simulink model "ActiveBalancingModelling"  (R2024b)
settings: Solver=FixedStepAuto  StartTime=0.0  StopTime=1000  FixedStep=SampleTime  RelTol=1e-3
model workspace (MAT data in the model file):
  Ah = 3
  C = 0.001
  R = 0.001
  SampleTime = 0.0001
  SoC1 = 60
  SoC2 = 70
  SoC3 = 50
  SoC4 = 80
  Vnom = 3.7
undefined symbols (not defined in the file or in its folder): Ion, Lithium
libraries: spsIdealSwitchLib x8, spsSeriesRLCBranchLib x5, spsBatteryLib x4, sps_lib x1
settings Model: Creator=MOHAMED  LastModifiedBy=MOHAMED

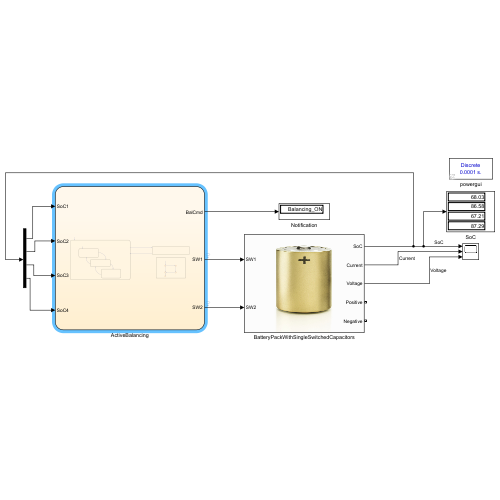
[thumbnail: Simulink's stored preview of the top-level diagram]
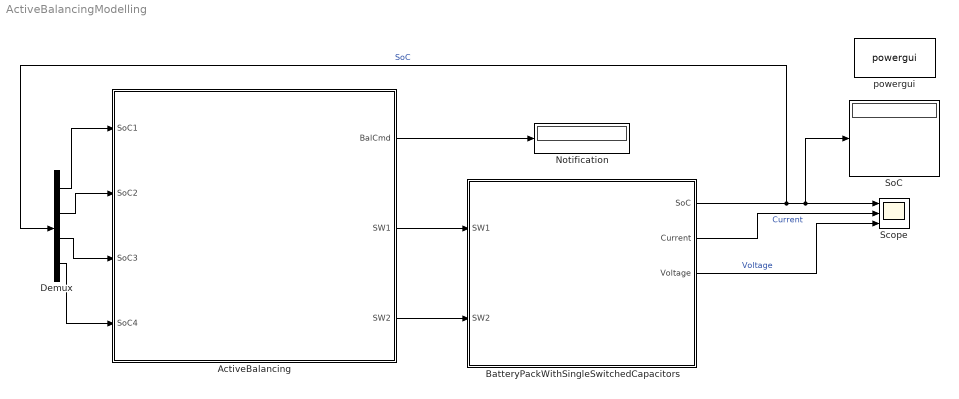
== system ActiveBalancingModelling ==
  ActiveBalancing : Stateflow chart  TreatAsAtomicUnit=on
  BatteryPackWithSingleSwitchedCapacitors : Subsystem
      mask Display: image('battery.jpg');
  Demux : Demux
  Notification : Display
  Scope : Scope  NumInputPorts=3
  SoC : Display
  powergui : sps_lib/powergui  Priority=1  SimulationMode=Discrete  SampleTime=SampleTime  frequency=60  Iterations=50  frequencyindice=0  Pbase=100e6  ErrMax=1e-4  UnitsV=kV  UnitsW=MW  buscounter=0  FunctionMessages=off  echomessages=off  EnableUseOfTLC=off  CurrentSourceSwitches=off  DisableSnubberDevices=off  DisableRonSwitches=off  DisableVfSwitches=off  DisplayEquations=off  AutomaticDiscreteSolvers=off  SolverType=Tustin/Backward Euler (TBE)  Interpol=off  ExternalGateDelay=off  methode=off  Ts=100  x0status=blocks  SPID=on  SwTol=0  HookPort=off  NonlinearTolerance=1e-4  nMaxIteration=100  ContinueOnMaxIteration=off  RestoreLinks=warning  ResistiveCurrentMeasurement=off  Frange=[0:2:500]  Ylog=off  Xlog=on  ShowGrid=off  save=off  variable=ZData  structure=0  ZoomFFT=off  StartTime=0.0  cycles=1  DisplayStyle=1  fundamental=60  FreqAxis=off  MaxFrequency=1000  frequencyindicesteady=1  RmsSteady=1  display=off
  wires:
  BatteryPackWithSingleSwitchedCapacitors/1(SoC) -> Demux/1, SoC/1, Scope/1  "SoC"
  BatteryPackWithSingleSwitchedCapacitors/2(Current) -> Scope/2  "Current"
  BatteryPackWithSingleSwitchedCapacitors/3(Voltage) -> Scope/3  "Voltage"
  ActiveBalancing/1(BalCmd) -> Notification/1
  ActiveBalancing/2(SW1) -> BatteryPackWithSingleSwitchedCapacitors/1(SW1)
  ActiveBalancing/3(SW2) -> BatteryPackWithSingleSwitchedCapacitors/2(SW2)
  Demux/1 -> ActiveBalancing/1(SoC1)
  Demux/2 -> ActiveBalancing/2(SoC2)
  Demux/3 -> ActiveBalancing/3(SoC3)
  Demux/4 -> ActiveBalancing/4(SoC4)

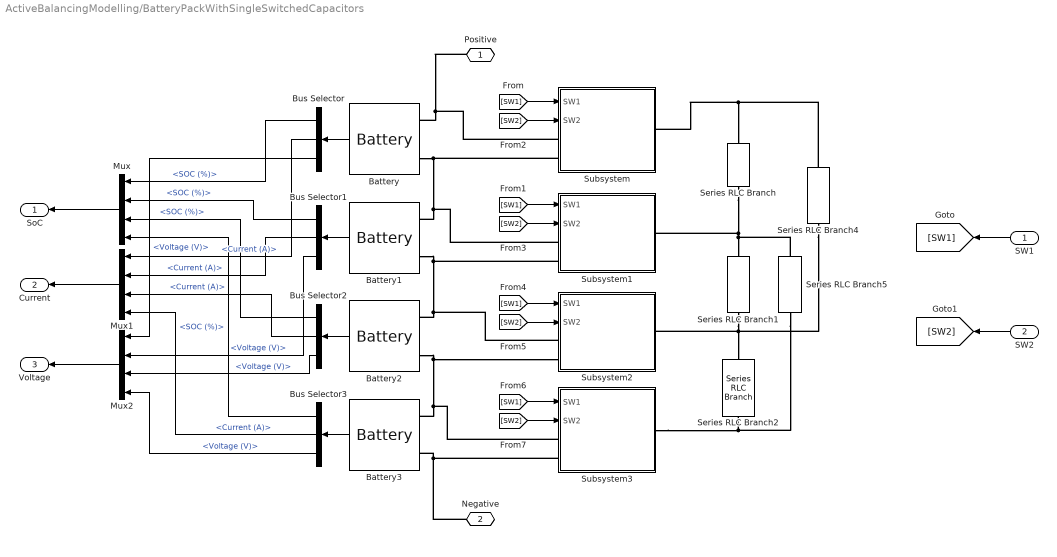
== system ActiveBalancingModelling/BatteryPackWithSingleSwitchedCapacitors ==
  SW1 : Inport
  SW2 : Inport  Port=2
  Battery : spsBatteryLib/Battery  BatType=Lithium-Ion  NomV=Vnom  NomQ=Ah  SOC=SoC1  Batt_Tr=20e-3  PresetModel=on  MaxQ=3  MinV=2.775  FullV=4.3068  Dis_rate=1.3043  R=0.012333  Normal_OP=2.713  expZone="[3.9974     0.14739]"
  Battery1 : spsBatteryLib/Battery  BatType=Lithium-Ion  NomV=Vnom  NomQ=Ah  SOC=SoC2  Batt_Tr=20e-3  PresetModel=on  MaxQ=3  MinV=2.775  FullV=4.3068  Dis_rate=1.3043  R=0.012333  Normal_OP=2.713  expZone="[3.9974     0.14739]"
  Battery2 : spsBatteryLib/Battery  BatType=Lithium-Ion  NomV=Vnom  NomQ=Ah  SOC=SoC3  Batt_Tr=20e-3  PresetModel=on  MaxQ=3  MinV=2.775  FullV=4.3068  Dis_rate=1.3043  R=0.012333  Normal_OP=2.713  expZone="[3.9974     0.14739]"
  Battery3 : spsBatteryLib/Battery  BatType=Lithium-Ion  NomV=Vnom  NomQ=Ah  SOC=SoC4  Batt_Tr=20e-3  PresetModel=on  MaxQ=3  MinV=2.775  FullV=4.3068  Dis_rate=1.3043  R=0.012333  Normal_OP=2.713  expZone="[3.9974     0.14739]"
  Bus Selector{,1..3} (4 alike) : BusSelector  OutputSignals=SOC (%),Current (A),Voltage (V)
  Mux : Mux
  Mux1 : Mux
  Mux2 : Mux
  Series RLC Branch{,1..2,4..5} (5 alike) : spsSeriesRLCBranchLib/Series RLC Branch  LConnTagsString=__new0  RConnTagsString=__new0  BranchType=C  Resistance=R  Inductance=1e-3  SetiL0=off  InitialCurrent=0  Capacitance=C  Setx0=off  InitialVoltage=0  Measurements=None
  Subsystem : Subsystem
  Subsystem1 : Subsystem
  Subsystem2 : Subsystem
  Subsystem3 : Subsystem
  Positive : PMIOPort  Side=Right
  Negative : PMIOPort  Port=2  Side=Right
  SoC : Outport
  Current : Outport  Port=2
  Voltage : Outport  Port=3
  wires:
  Mux1/1 -> Current/1
  Mux2/1 -> Voltage/1
  Mux/1 -> SoC/1
  Bus Selector3/3 -> Mux2/4  "<Voltage (V)>"
  Bus Selector2/3 -> Mux2/3  "<Voltage (V)>"
  Bus Selector/3 -> Mux2/1  "<Voltage (V)>"
  Bus Selector3/2 -> Mux1/4  "<Current (A)>"
  Bus Selector2/2 -> Mux1/3  "<Current (A)>"
  Bus Selector1/3 -> Mux2/2  "<Voltage (V)>"
  Bus Selector1/2 -> Mux1/2  "<Current (A)>"
  Bus Selector/2 -> Mux1/1  "<Current (A)>"
  Bus Selector3/1 -> Mux/4  "<SOC (%)>"
  Bus Selector2/1 -> Mux/3  "<SOC (%)>"
  Bus Selector1/1 -> Mux/2  "<SOC (%)>"
  Bus Selector/1 -> Mux/1  "<SOC (%)>"
  Battery2/1 -> Bus Selector2/1
  Battery3/1 -> Bus Selector3/1
  Battery1/1 -> Bus Selector1/1
  Battery/1 -> Bus Selector/1
  [SW1] -> Subsystem/1(SW1)
  [SW2] -> Subsystem/2(SW2)
  SW1/1 -> [SW1]
  SW2/1 -> [SW2]
  [SW2] -> Subsystem1/2(SW2)
  [SW1] -> Subsystem1/1(SW1)
  [SW1] -> Subsystem2/1(SW1)
  [SW2] -> Subsystem2/2(SW2)
  [SW2] -> Subsystem3/2(SW2)
  [SW1] -> Subsystem3/1(SW1)
  connections:
  Negative/RConn1 -- Subsystem3/LConn2 -- Battery3/LConn2
  Positive/RConn1 -- Battery/LConn1 -- Subsystem/LConn1
  Battery2/LConn2 -- Subsystem2/LConn2 -- Battery3/LConn1 -- Subsystem3/LConn1
  Battery1/LConn2 -- Battery2/LConn1 -- Subsystem2/LConn1 -- Subsystem1/LConn2
  Battery/LConn2 -- Battery1/LConn1 -- Subsystem1/LConn1 -- Subsystem/LConn2
  Series RLC Branch1/RConn1 -- Series RLC Branch2/LConn1 -- Series RLC Branch4/RConn1 -- Subsystem2/RConn1
  Subsystem3/RConn1 -- Series RLC Branch5/RConn1 -- Series RLC Branch2/RConn1
  Series RLC Branch4/LConn1 -- Series RLC Branch/LConn1 -- Subsystem/RConn1
  Series RLC Branch/RConn1 -- Series RLC Branch5/LConn1 -- Series RLC Branch1/LConn1 -- Subsystem1/RConn1

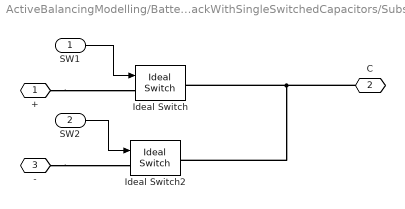
== system ActiveBalancingModelling/BatteryPackWithSingleSwitchedCapacitors/Subsystem ==
  SW1 : Inport
  SW2 : Inport  Port=2
  Ideal Switch : spsIdealSwitchLib/Ideal Switch  Ron=0.001  Lon=0  IC=0  Rs=1e5  Cs=inf  Measurements=off
  Ideal Switch2 : spsIdealSwitchLib/Ideal Switch  Ron=0.001  Lon=0  IC=0  Rs=1e5  Cs=inf  Measurements=off
  + : PMIOPort  Side=Left
  C : PMIOPort  Port=2  Side=Right
  - : PMIOPort  Port=3  Side=Left
  wires:
  SW2/1 -> Ideal Switch2/1
  SW1/1 -> Ideal Switch/1
  connections:
  -/RConn1 -- Ideal Switch2/LConn1
  C/RConn1 -- Ideal Switch/RConn1 -- Ideal Switch2/RConn1
  +/RConn1 -- Ideal Switch/LConn1

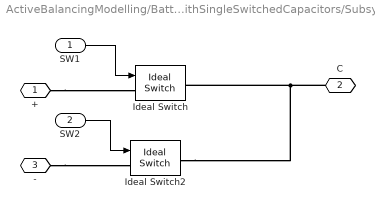
== system ActiveBalancingModelling/BatteryPackWithSingleSwitchedCapacitors/Subsystem1 ==
  SW1 : Inport
  SW2 : Inport  Port=2
  Ideal Switch : spsIdealSwitchLib/Ideal Switch  Ron=0.001  Lon=0  IC=0  Rs=1e5  Cs=inf  Measurements=off
  Ideal Switch2 : spsIdealSwitchLib/Ideal Switch  Ron=0.001  Lon=0  IC=0  Rs=1e5  Cs=inf  Measurements=off
  + : PMIOPort  Side=Left
  C : PMIOPort  Port=2  Side=Right
  - : PMIOPort  Port=3  Side=Left
  wires:
  SW1/1 -> Ideal Switch/1
  SW2/1 -> Ideal Switch2/1
  connections:
  +/RConn1 -- Ideal Switch/LConn1
  -/RConn1 -- Ideal Switch2/LConn1
  C/RConn1 -- Ideal Switch2/RConn1 -- Ideal Switch/RConn1

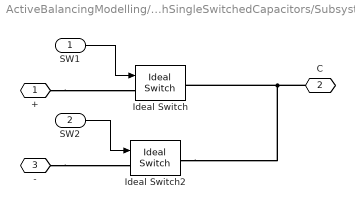
== system ActiveBalancingModelling/BatteryPackWithSingleSwitchedCapacitors/Subsystem2 ==
  SW1 : Inport
  SW2 : Inport  Port=2
  Ideal Switch : spsIdealSwitchLib/Ideal Switch  Ron=0.001  Lon=0  IC=0  Rs=1e5  Cs=inf  Measurements=off
  Ideal Switch2 : spsIdealSwitchLib/Ideal Switch  Ron=0.001  Lon=0  IC=0  Rs=1e5  Cs=inf  Measurements=off
  + : PMIOPort  Side=Left
  C : PMIOPort  Port=2  Side=Right
  - : PMIOPort  Port=3  Side=Left
  wires:
  SW2/1 -> Ideal Switch2/1
  SW1/1 -> Ideal Switch/1
  connections:
  -/RConn1 -- Ideal Switch2/LConn1
  C/RConn1 -- Ideal Switch/RConn1 -- Ideal Switch2/RConn1
  +/RConn1 -- Ideal Switch/LConn1

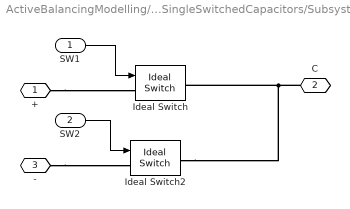
== system ActiveBalancingModelling/BatteryPackWithSingleSwitchedCapacitors/Subsystem3 ==
  SW1 : Inport
  SW2 : Inport  Port=2
  Ideal Switch : spsIdealSwitchLib/Ideal Switch  Ron=0.001  Lon=0  IC=0  Rs=1e5  Cs=inf  Measurements=off
  Ideal Switch2 : spsIdealSwitchLib/Ideal Switch  Ron=0.001  Lon=0  IC=0  Rs=1e5  Cs=inf  Measurements=off
  + : PMIOPort  Side=Left
  C : PMIOPort  Port=2  Side=Right
  - : PMIOPort  Port=3  Side=Left
  wires:
  SW1/1 -> Ideal Switch/1
  SW2/1 -> Ideal Switch2/1
  connections:
  +/RConn1 -- Ideal Switch/LConn1
  C/RConn1 -- Ideal Switch/RConn1 -- Ideal Switch2/RConn1
  -/RConn1 -- Ideal Switch2/LConn1

== stateflow chart ActiveBalancingModelling/ActiveBalancing ==
  state BalancingON
    en, du:
    BalCmd = Command.Balancing_ON;
    state SW1_Activation
      en, du:
      SW1 = 1;
      SW2 = 0;
      ex:
      flag = 1;
    state SignalDelay
      en, du:
      SW1 = 0;
      SW2 = 0;
    state SW2_Activation
      en, du:
      SW1 = 0;
      SW2 = 1;
      ex:
      flag = 0;
    (default) -> SW1_Activation
    SW1_Activation -> SignalDelay : after(0.45/frequency, sec)
    SignalDelay -> SW1_Activation [order 1] : after(0.05/frequency, sec)[flag == 0]
    SignalDelay -> SW2_Activation [order 2] : after(0.05/frequency, sec)[flag == 1]
    SW2_Activation -> SignalDelay : after(0.45/frequency, sec)
  state BalancingOFF
    en:
    BalCmd = Command.Balancing_OFF;
    SW1 = 0;
    SW2 = 0;
  state out = BalOFF(SoC1, SoC2, SoC3, SoC4) [function]
    (default) -> (junction 80)
    (junction 80) -> (junction 81) [order 1] : [abs(SoC1 - SoC2) > 0.001 ...
        | && abs(SoC1 - SoC3) > 0.001 ...
        | && abs(SoC1 - SoC4) > 0.001]
    (junction 80) -> (junction 82) [order 2] : {out = 1;}
    (junction 81) -> (junction 83) : {out = 0;}
    (junction 83) -> (junction 82)
    (junction 82) -> (junction 84)
  (default) -> BalancingON
  BalancingON -> BalancingOFF : [BalOFF(SoC1, SoC2, SoC3, SoC4)]
  BalancingOFF -> BalancingON : [~BalOFF(SoC1, SoC2, SoC3, SoC4)]
  data: SoC1 function_input; out function_output; SoC2 function_input; SoC3 function_input; SoC4 function_input; BalCmd output; SoC1 input; SW1 output; SW2 output; frequency local =1; SoC2 input; SoC3 input; SoC4 input; flag local
